simulink library "simulinkOSC_lib"  (R2018b)
settings: Solver=VariableStepAuto  StartTime=0.0  StopTime=10.0  RelTol=1e-3
settings Model: Creator=Ulysses  LastModifiedBy=Ulysses

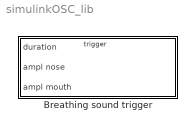
== system simulinkOSC_lib ==
  Breathing sound trigger : Subsystem  mask{server='localhost', port=57120, pathsyndefs='', pathwavs=''}
      mask prompts: pathsyndefs "Path syndefs"; pathwavs "Path wavs"
      mask TypeOptions server: simulinkOSC/server
      mask TypeOptions port: simulinkOSC/port
      mask TypeOptions pathsyndefs: simulinkOSC/pathsyndefs
      mask TypeOptions pathwavs: simulinkOSC/pathwavs
      mask Display:
      | port_label('input', 1, 'duration')
      | port_label('input', 2, 'ampl nose')
      | port_label('input', 3, 'ampl mouth')
      | disp(get_param(gcb,'server') + "\n" + get_param(gcb,'port'))

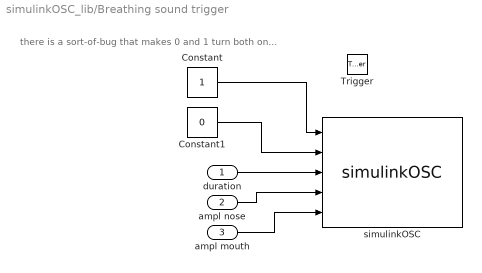
== system simulinkOSC_lib/Breathing sound trigger ==
  note: there is a sort-of-bug that makes 0 and 1 turn both on...
  duration : Inport
  ampl nose : Inport  Port=2
  ampl mouth : Inport  Port=3
  Trigger : TriggerPort  VariantControl=Variant  PortDimensions=1
  Constant : Constant
  Constant1 : Constant  Value=0
  simulinkOSC : S-Function  FunctionName=simulinkOSC  Parameters=uint16(server), uint16(port), uint16(pathsyndefs), uint16(pathwavs)  SFunctionDeploymentMode=off  EnableBusSupport=off  mask{server=server, port=port, pathsyndefs=pathsyndefs, pathwavs=pathwavs}
      mask prompts: pathsyndefs "Path syndefs"; pathwavs "Path wavs"
      mask Display:
      | port_label('input', 1, 'use nose')
      | port_label('input', 2, 'use mouth')
      | port_label('input', 3, 'duration')
      | port_label('input', 4, 'ampl nose')
      | port_label('input', 5, 'ampl mouth')
  wires:
  duration/1 -> simulinkOSC/3
  ampl mouth/1 -> simulinkOSC/5
  ampl nose/1 -> simulinkOSC/4
  Constant/1 -> simulinkOSC/1
  Constant1/1 -> simulinkOSC/2
